simulink model "cruise_open_loop_discrete"  (R2017a)
settings: Solver=VariableStepAuto  StartTime=0.0  StopTime=700  RelTol=1e-3
settings Model: Creator=root  LastModifiedBy=root

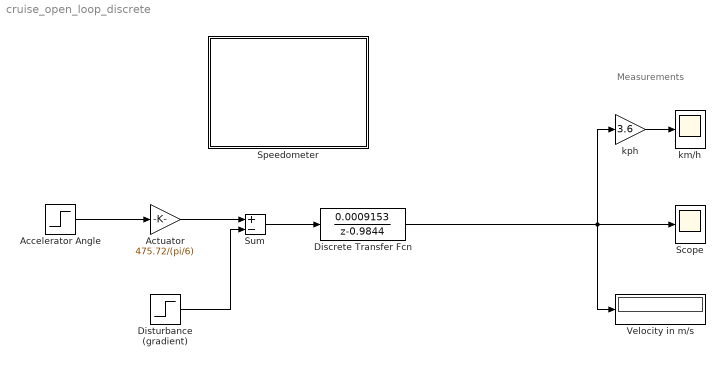
== system cruise_open_loop_discrete ==
  note: Measurements
  Accelerator Angle : Step  After=pi/6  SampleTime=0
  Actuator : Gain  Gain=475.72/(pi/6)
  Discrete Transfer Fcn : DiscreteTransferFcn  Numerator=[0.0009153]  Denominator=[1 -0.9844]  SampleTime=1
  Disturbance (gradient) : Step  Time=800  After=475.72*9.81*sin(pi/45)  SampleTime=0
  Scope : Scope
  Speedometer : Subsystem  DialogController=hmiCreateDDGDialog  IsWebBlock=on  mask(MWDashboardBlock){webBlockId=c77fd51c-fd22-40a0-8bec-fa9513db74d2, webBlockType=semicirculargauge, ShowInLibBrowser=on, ShowInitialText=on, HMISrcModelName=cruise_open_loop_discrete}
      mask prompts: webBlockId "WebBlock Id"; webBlockType "WebBlock Type"; HMISrcModelName "Source Model"
      mask help: SimulinkHMI:dialogs:SemicircularGaugeDialogDesc
      mask Help: helpview([docroot '/mapfiles/simulink.map'], 'hmi_half_gauge')
      mask Display:
      | if strcmp(get_param(bdroot(gcb),'BlockDiagramType'), 'library')
      |     image([(matlabroot) '/toolbox/simulink/hmi/icons/SemicircularGauge.png']);
      | end
  Sum : Sum  Inputs=+-
  Velocity in m/s : Display
  km/h : Scope
  kph : Gain  Gain=3.6
  wires:
  Discrete Transfer Fcn/1 -> kph/1, Velocity in m/s/1, Scope/1
  Disturbance (gradient)/1 -> Sum/2
  Actuator/1 -> Sum/1
  Sum/1 -> Discrete Transfer Fcn/1
  Accelerator Angle/1 -> Actuator/1
  kph/1 -> km/h/1

== system cruise_open_loop_discrete/Speedometer ==
